simulink model "Mrac_IeI"  (R2021a)
settings: Solver=VariableStepAuto  StartTime=0.0  StopTime=50  RelTol=1e-3
settings Model: Creator=simon  LastModifiedBy=simon

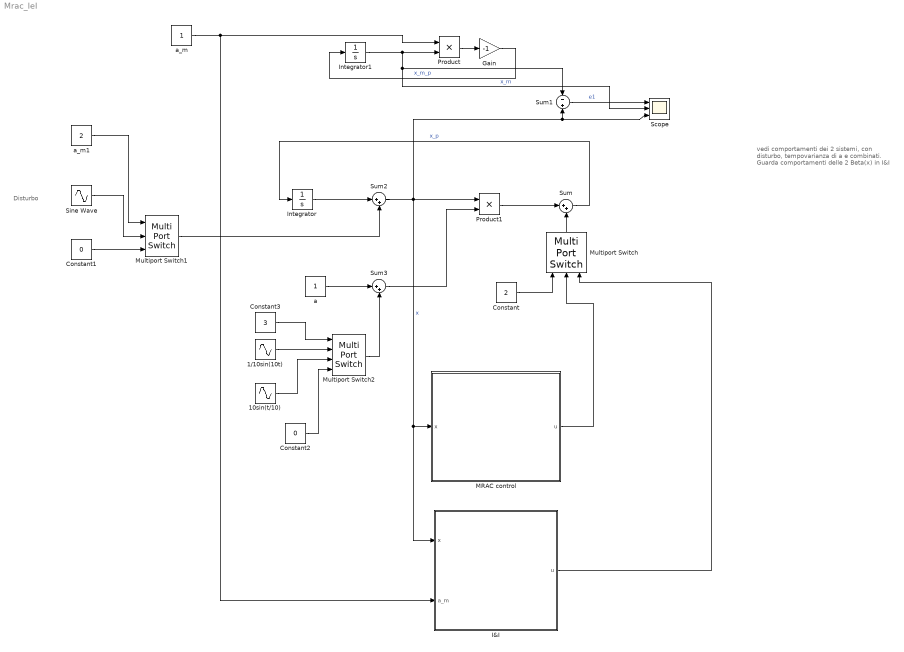
== system Mrac_IeI ==
  note: vedi comportamenti dei 2 sistemi, con
      | disturbo, tempovarianza di a e combinati.
      | Guarda comportamenti delle 2 Beta(x)
      | in I&I
  note: Disturbo
  1/10sin(10t) : Sin  Amplitude=1/10  Frequency=10  SampleTime=0
  10sin(t/10) : Sin  Amplitude=10  Frequency=1/10  SampleTime=0
  Constant : Constant  Value=2
  Constant1 : Constant  Value=0
  Constant2 : Constant  Value=0
  Constant3 : Constant  Value=3
  Gain : Gain  Gain=-1
  I&I : Subsystem
  Integrator : Integrator  InitialCondition=2
  Integrator1 : Integrator  InitialCondition=2
  MRAC control : Subsystem
  Multiport Switch : MultiPortSwitch  Inputs=2
  Multiport Switch1 : MultiPortSwitch  Inputs=2
  Multiport Switch2 : MultiPortSwitch
  Product : Product
  Product1 : Product
  Scope : Scope  NumInputPorts=3
  Sine Wave : Sin  Amplitude=0.1  Frequency=1/5  SampleTime=0
  Sum : Sum  Inputs=|++
  Sum1 : Sum  Inputs=-+
  Sum2 : Sum  Inputs=|++
  Sum3 : Sum  Inputs=|++
  a : Constant
  a_m : Constant
  a_m1 : Constant  Value=2
  wires:
  Product1/1 -> Sum/1
  Sum/1 -> Integrator/1  "x_p"
  Integrator1/1 -> Scope/2, Sum1/1, Product/2  "x_m"
  Gain/1 -> Integrator1/1  "x_m_p"
  Sum1/1 -> Scope/1  "e1"
  Multiport Switch/1 -> Sum/2
  MRAC control/1(u) -> Multiport Switch/2
  Constant/1 -> Multiport Switch/1
  Product/1 -> Gain/1
  a_m/1 -> Product/1, I&I/2(a_m)
  I&I/1(u) -> Multiport Switch/3
  Sum2/1 -> Scope/3, Sum1/2, I&I/1(x), MRAC control/1(x), Product1/1  "x"
  Constant1/1 -> Multiport Switch1/3
  Sine Wave/1 -> Multiport Switch1/2
  a_m1/1 -> Multiport Switch1/1
  Multiport Switch1/1 -> Sum2/2
  Integrator/1 -> Sum2/1
  Sum3/1 -> Product1/2
  a/1 -> Sum3/1
  Constant2/1 -> Multiport Switch2/4
  Constant3/1 -> Multiport Switch2/1
  Multiport Switch2/1 -> Sum3/2
  1/10sin(10t)/1 -> Multiport Switch2/2
  10sin(t/10)/1 -> Multiport Switch2/3

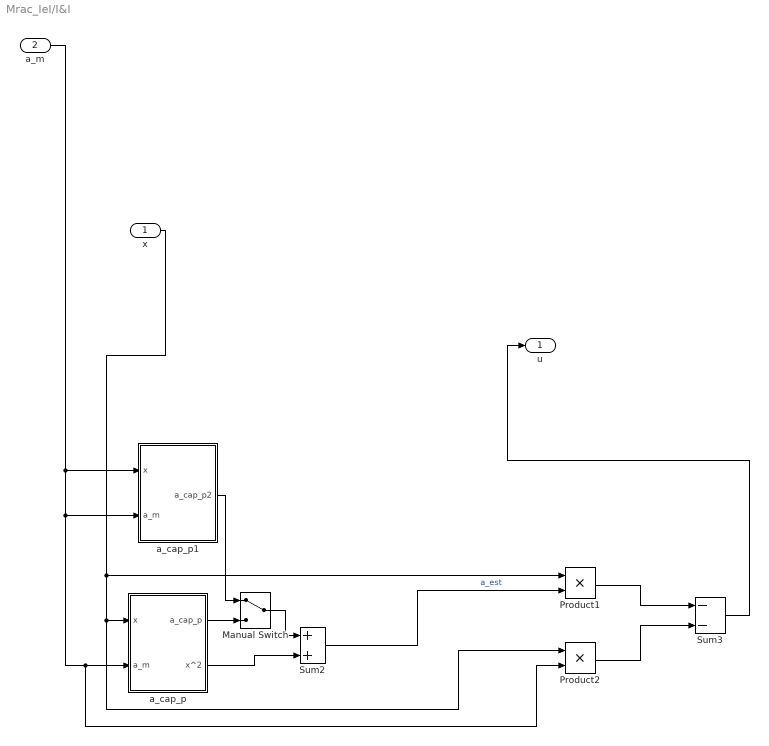
== system Mrac_IeI/I&I ==
  x : Inport
  a_m : Inport  Port=2
  Manual Switch : ManualSwitch
  Product1 : Product
  Product2 : Product
  Sum2 : Sum
  Sum3 : Sum  Inputs=--
  a_cap_p : Subsystem
  a_cap_p1 : Subsystem
  u : Outport
  wires:
  Product2/1 -> Sum3/2
  a_cap_p/2(x^2) -> Sum2/2
  Sum2/1 -> Product1/2  "a_est"
  Product1/1 -> Sum3/1
  Sum3/1 -> u/1
  a_m/1 -> a_cap_p1/1(x), a_cap_p1/2(a_m), Product2/2, a_cap_p/2(a_m)
  x/1 -> Product1/1, a_cap_p/1(x), Product2/1
  a_cap_p/1(a_cap_p) -> Manual Switch/2
  Manual Switch/1 -> Sum2/1
  a_cap_p1/1(a_cap_p2) -> Manual Switch/1

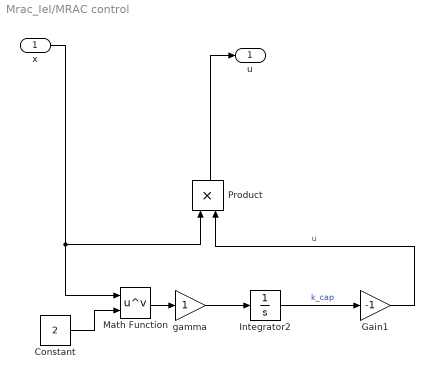
== system Mrac_IeI/MRAC control ==
  x : Inport
  Constant : Constant  Value=2
  Gain1 : Gain  Gain=-1
  Integrator2 : Integrator  InitialCondition=1
  Math Function : Math  Operator=pow  SaturateOnIntegerOverflow=on
  Product : Product
  gamma : Gain
  u : Outport
  wires:
  Math Function/1 -> gamma/1
  Constant/1 -> Math Function/2
  Integrator2/1 -> Gain1/1  "k_cap"
  gamma/1 -> Integrator2/1
  x/1 -> Product/1, Math Function/1
  Gain1/1 -> Product/2  "u"
  Product/1 -> u/1

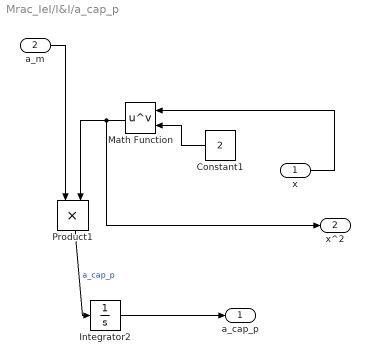
== system Mrac_IeI/I&I/a_cap_p ==
  x : Inport
  a_m : Inport  Port=2
  Constant1 : Constant  Value=2
  Integrator2 : Integrator
  Math Function : Math  Operator=pow  SaturateOnIntegerOverflow=on
  Product1 : Product
  a_cap_p : Outport
  x^2 : Outport  Port=2
  wires:
  Math Function/1 -> x^2/1, Product1/2
  Constant1/1 -> Math Function/2
  a_m/1 -> Product1/1
  Integrator2/1 -> a_cap_p/1
  Product1/1 -> Integrator2/1  "a_cap_p"
  x/1 -> Math Function/1

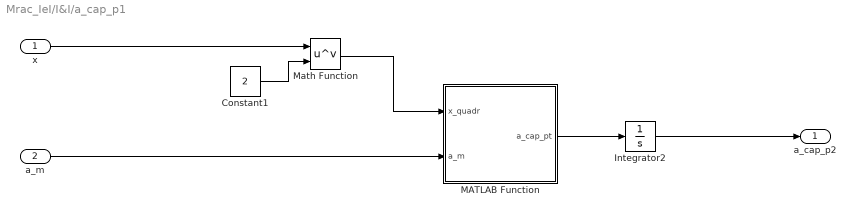
== system Mrac_IeI/I&I/a_cap_p1 ==
  x : Inport
  a_m : Inport  Port=2
  Constant1 : Constant  Value=2
  Integrator2 : Integrator
  MATLAB Function : MATLAB Function  TreatAsAtomicUnit=on
  Math Function : Math  Operator=pow  SaturateOnIntegerOverflow=on
  a_cap_p2 : Outport
  wires:
  Math Function/1 -> MATLAB Function/1(x_quadr)
  Constant1/1 -> Math Function/2
  a_m/1 -> MATLAB Function/2(a_m)
  Integrator2/1 -> a_cap_p2/1
  x/1 -> Math Function/1
  MATLAB Function/1(a_cap_pt) -> Integrator2/1

== matlab function Mrac_IeI/I&I/a_cap_p1/MATLAB Function ==
  data: x_quadr input; a_m input; a_cap_pt output
function a_cap_pt = fcn(x_quadr, a_m)

a_cap_pt = (a_m*x_quadr)/(1+x_quadr);
